simulink model "c_Simulink_Maglev_Tower_lift_motion_control"  (R2020a)
settings: Solver=ode1  StartTime=0.0  StopTime=1  FixedStep=dt  RelTol=1e-3
InitFcn:
  | %parameters_Maglev_Tower_lift_motion
values from neighbouring files (symbols this model uses):
  A1 = -2*r*cos(w0)    [a_system_response_continuous.m]    (also in a_system_response_discrete.m; b_parameters_Maglev_Tower_lift_motion.m)
  A2 = r*r    (= 0.9801)    [a_system_response_continuous.m]    (also in a_system_response_discrete.m; b_parameters_Maglev_Tower_lift_motion.m)
  b = 2*pi*1    (= 6.28318530718)    [a_system_response_continuous.m]    (also in a_system_response_discrete.m; b_parameters_Maglev_Tower_lift_motion.m = 0)
  B0 = 1    [a_system_response_continuous.m]    (also in a_system_response_discrete.m; b_parameters_Maglev_Tower_lift_motion.m)
  B1 = -2*cos(w0)    [a_system_response_continuous.m]    (also in a_system_response_discrete.m; b_parameters_Maglev_Tower_lift_motion.m)
  B2 = 1    [a_system_response_continuous.m]    (also in a_system_response_discrete.m; b_parameters_Maglev_Tower_lift_motion.m)
  d = dt/(dt+2*tau_current)    (= 0.0591173974417)    [a_system_response_discrete.m]    (also in b_parameters_Maglev_Tower_lift_motion.m = 0.12947)
  dpitch_ref_frequency = 2*pi*0.5    (= 3.14159265359)    [b_parameters_Maglev_Tower_lift_motion.m]
  dpitch_ref_mag = 0.001    [b_parameters_Maglev_Tower_lift_motion.m]
  droll_ref_frequency = 2*pi*0.1    (= 0.628318530718)    [b_parameters_Maglev_Tower_lift_motion.m]
  droll_ref_mag = 0.001    [b_parameters_Maglev_Tower_lift_motion.m]
  dt = 1/5000    (= 0.0002)    [a_system_response_discrete.m]    (also in b_parameters_Maglev_Tower_lift_motion.m)
  dx_ref_frequency = 2*pi*5    (= 31.4159265359)    [b_parameters_Maglev_Tower_lift_motion.m]
  dx_ref_mag = 0.001    [b_parameters_Maglev_Tower_lift_motion.m]
  dy_ref_frequency = 2*pi*10    (= 62.8318530718)    [b_parameters_Maglev_Tower_lift_motion.m]
  dy_ref_mag = 0.001    [b_parameters_Maglev_Tower_lift_motion.m]
  dyaw_ref_frequency = 2*pi*1    (= 6.28318530718)    [b_parameters_Maglev_Tower_lift_motion.m]
  dyaw_ref_mag = 0.001    [b_parameters_Maglev_Tower_lift_motion.m]
  h = 327.07 * 1e-3    (= 0.32707)    [b_parameters_Maglev_Tower_lift_motion.m]
  ha = 373.57 * 1e-3    (= 0.37357)    [b_parameters_Maglev_Tower_lift_motion.m]
  isnoise = 1    [b_parameters_Maglev_Tower_lift_motion.m]
  Ix = Ix_cg    (= 41.394)    [b_parameters_Maglev_Tower_lift_motion.m]
  Iy = Iy_cg + M*da^2    (= 47.4067057344)    [b_parameters_Maglev_Tower_lift_motion.m]
  Iz = Iz_cg + M*da^2    (= 31.5217057344)    [b_parameters_Maglev_Tower_lift_motion.m]
  kc_current = 1    [b_parameters_Maglev_Tower_lift_motion.m]
  ki_current = 1    [b_parameters_Maglev_Tower_lift_motion.m]
  ki_pitch = ki    (= 500)    [b_parameters_Maglev_Tower_lift_motion.m]    (also in c_main_Maglev_Tower_lift_motion_control.m = ki_pitch*dt)
  ki_roll = ki    (= 500)    [b_parameters_Maglev_Tower_lift_motion.m]    (also in c_main_Maglev_Tower_lift_motion_control.m = ki_roll*dt)
  ki_x = ki    (= 500)    [b_parameters_Maglev_Tower_lift_motion.m]    (also in c_main_Maglev_Tower_lift_motion_control.m = ki_x*dt)
  ki_y = ki    (= 500)    [b_parameters_Maglev_Tower_lift_motion.m]    (also in c_main_Maglev_Tower_lift_motion_control.m = ki_y*dt)
  ki_yaw = ki    (= 500)    [b_parameters_Maglev_Tower_lift_motion.m]    (also in c_main_Maglev_Tower_lift_motion_control.m = ki_yaw*dt)
  kp_pitch = kp    (= 0.5)    [b_parameters_Maglev_Tower_lift_motion.m]    (also in c_main_Maglev_Tower_lift_motion_control.m = kp_pitch*dt)
  kp_roll = kp    (= 0.5)    [b_parameters_Maglev_Tower_lift_motion.m]    (also in c_main_Maglev_Tower_lift_motion_control.m = kp_roll*dt)
  kp_x = kp    (= 0.5)    [b_parameters_Maglev_Tower_lift_motion.m]    (also in c_main_Maglev_Tower_lift_motion_control.m = kp_x*dt)
  kp_y = kp    (= 0.5)    [b_parameters_Maglev_Tower_lift_motion.m]    (also in c_main_Maglev_Tower_lift_motion_control.m = kp_y*dt)
  kp_yaw = kp    (= 0.5)    [b_parameters_Maglev_Tower_lift_motion.m]    (also in c_main_Maglev_Tower_lift_motion_control.m = kp_yaw*dt)
  M = 302.667    [b_parameters_Maglev_Tower_lift_motion.m]
  pBu = pinv(Bu)    [b_parameters_Maglev_Tower_lift_motion.m]
  select_current_filter = 3    [b_parameters_Maglev_Tower_lift_motion.m]
  tau = 1/(2*pi*100)    (= 0.00159154943092)    [a_system_response_continuous.m]    (also in a_system_response_discrete.m; b_parameters_Maglev_Tower_lift_motion.m)
  tau_current = 1/(2*pi*100)    (= 0.00159154943092)    [a_system_response_continuous.m]    (also in a_system_response_discrete.m; b_parameters_Maglev_Tower_lift_motion.m)
  w = 219.77 * 1e-3    (= 0.21977)    [b_parameters_Maglev_Tower_lift_motion.m]
  w_current = 2*pi*5    (= 31.4159265359)    [a_system_response_continuous.m]    (also in a_system_response_discrete.m; b_parameters_Maglev_Tower_lift_motion.m)
  wa = 140.52 * 1e-3    (= 0.14052)    [b_parameters_Maglev_Tower_lift_motion.m]
  zeta = 0.707    [a_system_response_continuous.m]    (also in a_system_response_discrete.m; b_parameters_Maglev_Tower_lift_motion.m)
libraries: simulink x8
settings Model: Creator=JSPark  LastModifiedBy=JSPark
settings SolverCC: AlgebraicLoopSolver=LineSearch

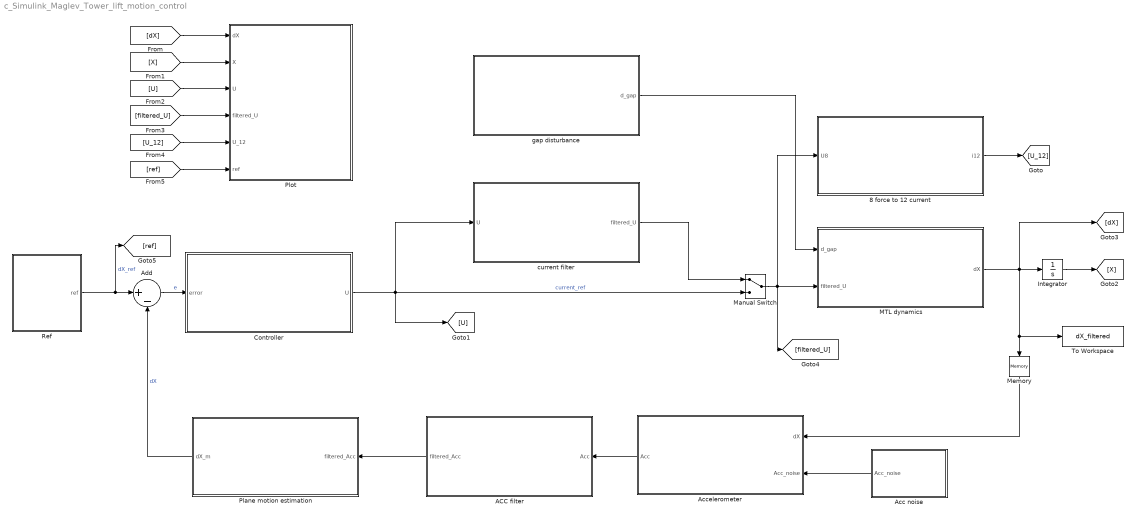
== system c_Simulink_Maglev_Tower_lift_motion_control ==
  8 force to 12 current : Subsystem
  ACC filter : Subsystem
  Acc noise : Subsystem
  Accelerometer : Subsystem
  Add : Sum  Inputs=|+-
  Controller : Subsystem
  Integrator : Integrator
  MTL dynamics : Subsystem
  Manual Switch : ManualSwitch
  Memory : Memory
  Plane motion estimation : Subsystem
  Plot : Subsystem
  Ref : Subsystem
  To Workspace : ToWorkspace  VariableName=dX_filtered  SampleTime=-1
  current filter : Subsystem
  gap disturbance : Subsystem
  wires:
  MTL dynamics/1(dX) -> [dX], To Workspace/1, Memory/1, Integrator/1
  Ref/1(ref) -> [ref], Add/1  "dX_ref"
  Plane motion estimation/1(dX_m) -> Add/2  "dX"
  Add/1 -> Controller/1(error)  "e"
  Accelerometer/1(Acc) -> ACC filter/1(Acc)
  Memory/1 -> Accelerometer/1(dX)
  Acc noise/1(Acc_noise) -> Accelerometer/2(Acc_noise)
  ACC filter/1(filtered_Acc) -> Plane motion estimation/1(filtered_Acc)
  Controller/1(U) -> [U], Manual Switch/2, current filter/1(U)  "current_ref"
  gap disturbance/1(d_gap) -> MTL dynamics/1(d_gap)
  Manual Switch/1 -> 8 force to 12 current/1(U8), [filtered_U], MTL dynamics/2(filtered_U)
  current filter/1(filtered_U) -> Manual Switch/1
  8 force to 12 current/1(i12) -> [U_12]
  Integrator/1 -> [X]
  [dX] -> Plot/1(dX)
  [X] -> Plot/2(X)
  [U] -> Plot/3(U)
  [filtered_U] -> Plot/4(filtered_U)
  [U_12] -> Plot/5(U_12)
  [ref] -> Plot/6(ref)

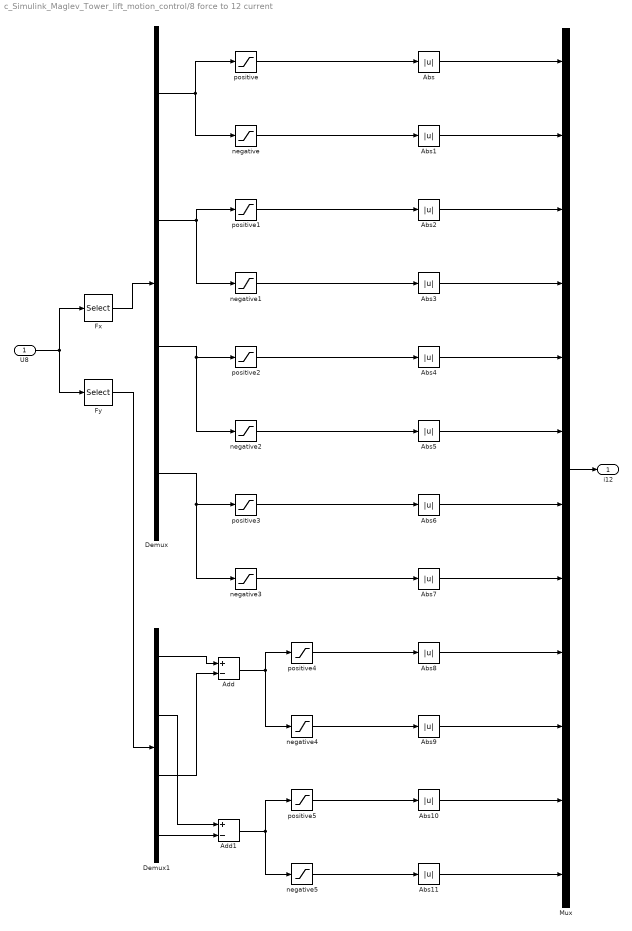
== system c_Simulink_Maglev_Tower_lift_motion_control/8 force to 12 current ==
  U8 : Inport
  Abs{,1..11} (12 alike) : Abs
  Add : Sum  Inputs=+-
  Add1 : Sum  Inputs=+-
  Demux : Demux
  Demux1 : Demux
  Fx : Selector  InputPortWidth=8  IndexOptions=Index vector (dialog)  Indices=[1:4]  OutputSizes=1
  Fy : Selector  InputPortWidth=8  IndexOptions=Index vector (dialog)  Indices=[5:8]  OutputSizes=1
  Mux : Mux  Inputs=12
  negative{,1..5} (6 alike) : Saturate  UpperLimit=0  LowerLimit=-100000
  positive{,1..5} (6 alike) : Saturate  UpperLimit=100000  LowerLimit=0
  i12 : Outport
  wires:
  U8/1 -> Fy/1, Fx/1
  Fx/1 -> Demux/1
  Demux/1 -> negative/1, positive/1
  positive/1 -> Abs/1
  negative/1 -> Abs1/1
  Demux/2 -> negative1/1, positive1/1
  positive1/1 -> Abs2/1
  negative1/1 -> Abs3/1
  positive2/1 -> Abs4/1
  negative2/1 -> Abs5/1
  positive3/1 -> Abs6/1
  negative3/1 -> Abs7/1
  Demux/3 -> negative2/1, positive2/1
  Demux/4 -> positive3/1, negative3/1
  Fy/1 -> Demux1/1
  Demux1/1 -> Add/1
  Demux1/3 -> Add/2
  Demux1/2 -> Add1/1
  Demux1/4 -> Add1/2
  Add/1 -> positive4/1, negative4/1
  Add1/1 -> positive5/1, negative5/1
  positive4/1 -> Abs8/1
  negative4/1 -> Abs9/1
  positive5/1 -> Abs10/1
  negative5/1 -> Abs11/1
  Mux/1 -> i12/1
  Abs/1 -> Mux/1
  Abs1/1 -> Mux/2
  Abs2/1 -> Mux/3
  Abs3/1 -> Mux/4
  Abs4/1 -> Mux/5
  Abs5/1 -> Mux/6
  Abs6/1 -> Mux/7
  Abs7/1 -> Mux/8
  Abs8/1 -> Mux/9
  Abs9/1 -> Mux/10
  Abs10/1 -> Mux/11
  Abs11/1 -> Mux/12

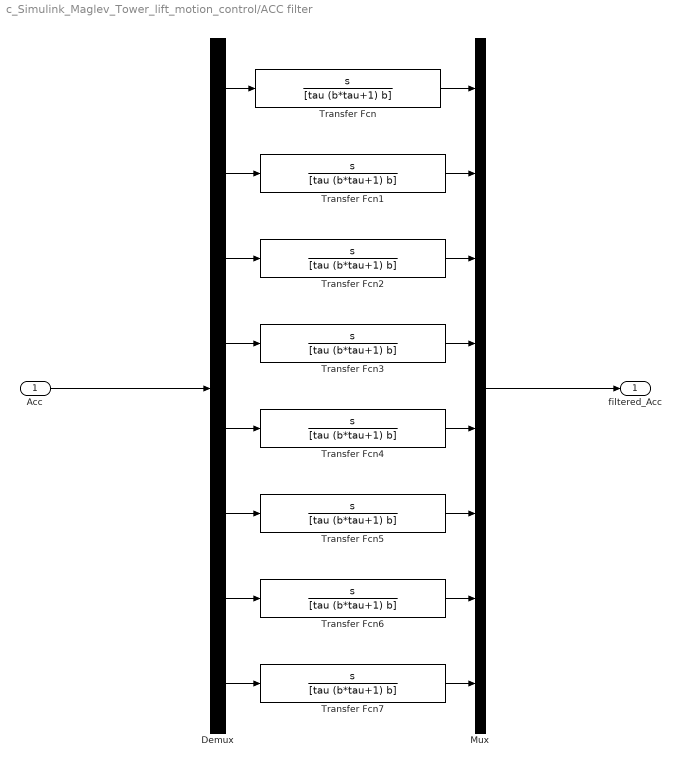
== system c_Simulink_Maglev_Tower_lift_motion_control/ACC filter ==
  Acc : Inport
  Demux : Demux  Outputs=8
  Mux : Mux  Inputs=8
  Transfer Fcn{,1..7} (8 alike) : TransferFcn  Numerator=[1 0]  Denominator=[tau (b*tau+1) b]
  filtered_Acc : Outport
  wires:
  Acc/1 -> Demux/1
  Demux/1 -> Transfer Fcn/1
  Demux/2 -> Transfer Fcn1/1
  Demux/3 -> Transfer Fcn2/1
  Demux/4 -> Transfer Fcn3/1
  Demux/5 -> Transfer Fcn4/1
  Demux/6 -> Transfer Fcn5/1
  Demux/7 -> Transfer Fcn6/1
  Demux/8 -> Transfer Fcn7/1
  Transfer Fcn/1 -> Mux/1
  Transfer Fcn1/1 -> Mux/2
  Transfer Fcn2/1 -> Mux/3
  Transfer Fcn3/1 -> Mux/4
  Transfer Fcn4/1 -> Mux/5
  Transfer Fcn5/1 -> Mux/6
  Transfer Fcn6/1 -> Mux/7
  Transfer Fcn7/1 -> Mux/8
  Mux/1 -> filtered_Acc/1

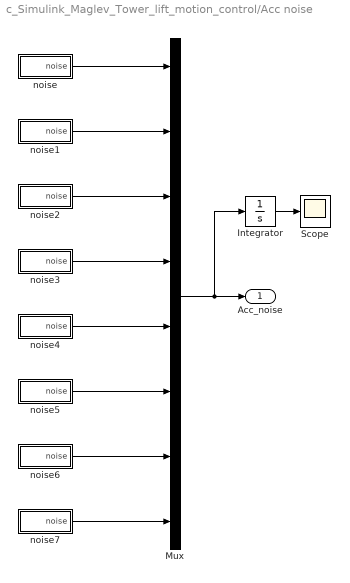
== system c_Simulink_Maglev_Tower_lift_motion_control/Acc noise ==
  Integrator : Integrator
  Mux : Mux  Inputs=8
  Scope : Scope
  noise : Subsystem
  noise1 : Subsystem
  noise2 : Subsystem
  noise3 : Subsystem
  noise4 : Subsystem
  noise5 : Subsystem
  noise6 : Subsystem
  noise7 : Subsystem
  Acc_noise : Outport
  wires:
  noise3/1(noise) -> Mux/4
  noise6/1(noise) -> Mux/7
  noise5/1(noise) -> Mux/6
  noise7/1(noise) -> Mux/8
  noise2/1(noise) -> Mux/3
  noise1/1(noise) -> Mux/2
  noise/1(noise) -> Mux/1
  noise4/1(noise) -> Mux/5
  Mux/1 -> Integrator/1, Acc_noise/1
  Integrator/1 -> Scope/1

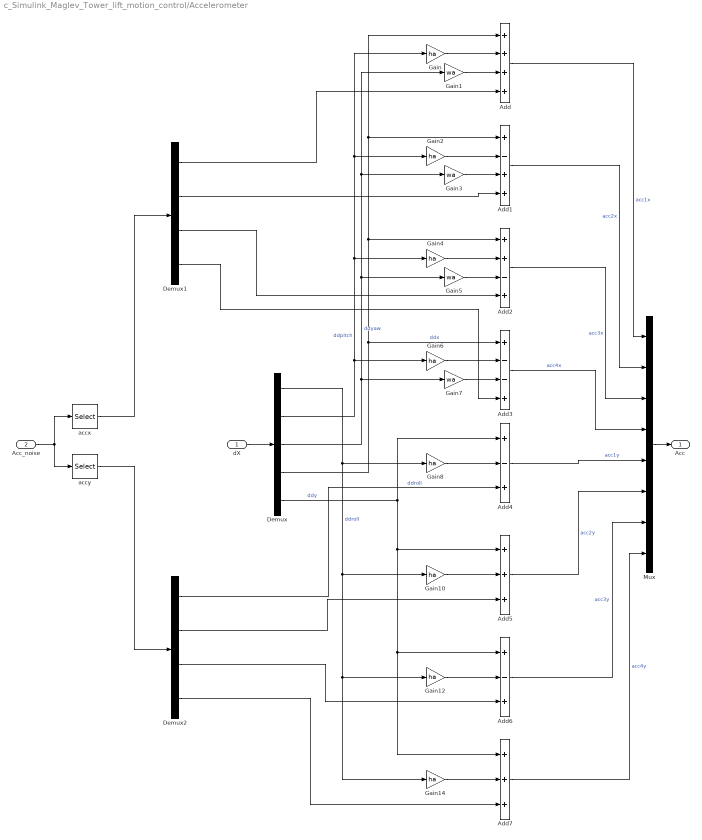
== system c_Simulink_Maglev_Tower_lift_motion_control/Accelerometer ==
  dX : Inport
  Acc_noise : Inport  Port=2
  Add : Sum  Inputs=++++
  Add1 : Sum  Inputs=+-++
  Add2 : Sum  Inputs=++-+
  Add3 : Sum  Inputs=+--+
  Add4 : Sum  Inputs=+-+
  Add5 : Sum  Inputs=+++
  Add6 : Sum  Inputs=+-+
  Add7 : Sum  Inputs=+++
  Demux : Demux  Outputs=5
  Demux1 : Demux
  Demux2 : Demux
  Gain{,2,4,6,8,10,12,14} (8 alike) : Gain  Gain=ha
  Gain{1,3,5,7} (4 alike) : Gain  Gain=wa
  Mux : Mux  Inputs=8
  accx : Selector  InputPortWidth=8  IndexOptions=Index vector (dialog)  Indices=[1:4]  OutputSizes=1
  accy : Selector  InputPortWidth=8  IndexOptions=Index vector (dialog)  Indices=[5:8]  OutputSizes=1
  Acc : Outport
  wires:
  Mux/1 -> Acc/1
  Demux/4 -> Add3/1, Add2/1, Add1/1, Add/1  "ddx"
  Demux/2 -> Gain6/1, Gain4/1, Gain2/1, Gain/1  "ddpitch"
  Demux/3 -> Gain7/1, Gain5/1, Gain3/1, Gain1/1  "ddyaw"
  Gain/1 -> Add/2
  Gain1/1 -> Add/3
  Add/1 -> Mux/1  "acc1x"
  Gain3/1 -> Add1/3
  Gain2/1 -> Add1/2
  Add1/1 -> Mux/2  "acc2x"
  Gain4/1 -> Add2/2
  Gain5/1 -> Add2/3
  Add2/1 -> Mux/3  "acc3x"
  Gain7/1 -> Add3/3
  Gain6/1 -> Add3/2
  Demux1/4 -> Add3/4
  Add3/1 -> Mux/4  "acc4x"
  Gain10/1 -> Add5/2
  Add4/1 -> Mux/5  "acc1y"
  Add7/1 -> Mux/8  "acc4y"
  Add6/1 -> Mux/7  "acc3y"
  Gain12/1 -> Add6/2
  Gain14/1 -> Add7/2
  Add5/1 -> Mux/6  "acc2y"
  Gain8/1 -> Add4/2
  Demux/5 -> Add5/1, Add6/1, Add7/1, Add4/1  "ddy"
  Demux/1 -> Gain8/1, Gain10/1, Gain12/1, Gain14/1  "ddroll"
  Demux2/2 -> Add5/3
  Demux2/3 -> Add6/3
  Demux2/4 -> Add7/3
  dX/1 -> Demux/1
  Acc_noise/1 -> accy/1, accx/1
  Demux1/1 -> Add/4
  Demux1/2 -> Add1/4
  Demux1/3 -> Add2/4
  Demux2/1 -> Add4/3  "ddroll"
  accx/1 -> Demux1/1
  accy/1 -> Demux2/1

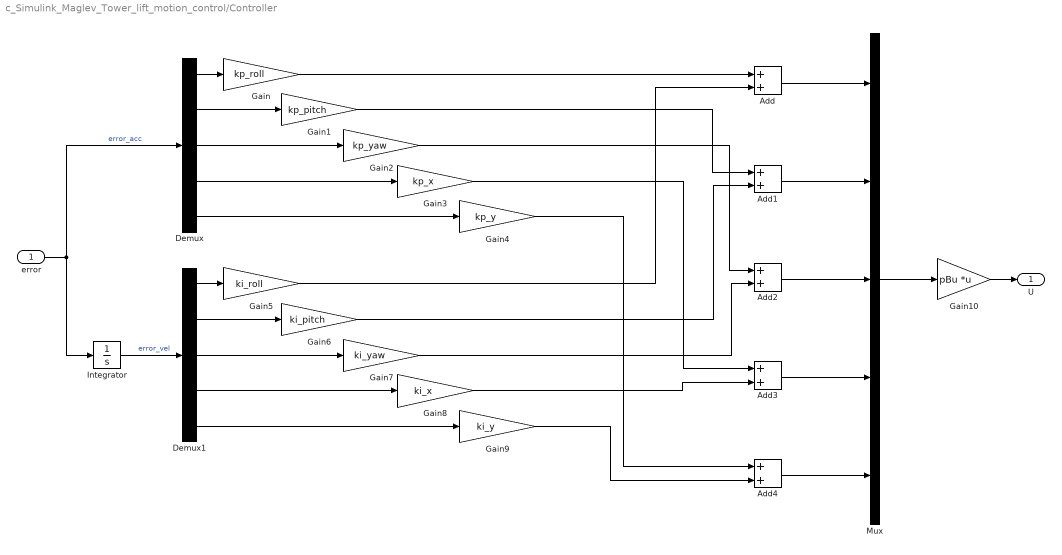
== system c_Simulink_Maglev_Tower_lift_motion_control/Controller ==
  error : Inport
  Add{,1..4} (5 alike) : Sum
  Demux : Demux  Outputs=5
  Demux1 : Demux  Outputs=5
  Gain : Gain  Gain=kp_roll
  Gain1 : Gain  Gain=kp_pitch
  Gain10 : Gain  Gain=pBu  Multiplication=Matrix(K*u)
  Gain2 : Gain  Gain=kp_yaw
  Gain3 : Gain  Gain=kp_x
  Gain4 : Gain  Gain=kp_y
  Gain5 : Gain  Gain=ki_roll
  Gain6 : Gain  Gain=ki_pitch
  Gain7 : Gain  Gain=ki_yaw
  Gain8 : Gain  Gain=ki_x
  Gain9 : Gain  Gain=ki_y
  Integrator : Integrator
  Mux : Mux  Inputs=5
  U : Outport
  wires:
  error/1 -> Integrator/1, Demux/1  "error_acc"
  Integrator/1 -> Demux1/1  "error_vel"
  Demux/1 -> Gain/1
  Demux/2 -> Gain1/1
  Demux/3 -> Gain2/1
  Demux/4 -> Gain3/1
  Demux/5 -> Gain4/1
  Demux1/3 -> Gain7/1
  Demux1/2 -> Gain6/1
  Demux1/5 -> Gain9/1
  Demux1/4 -> Gain8/1
  Demux1/1 -> Gain5/1
  Gain/1 -> Add/1
  Gain5/1 -> Add/2
  Gain1/1 -> Add1/1
  Gain6/1 -> Add1/2
  Gain2/1 -> Add2/1
  Gain7/1 -> Add2/2
  Gain3/1 -> Add3/1
  Gain8/1 -> Add3/2
  Gain4/1 -> Add4/1
  Gain9/1 -> Add4/2
  Add/1 -> Mux/1
  Add1/1 -> Mux/2
  Add2/1 -> Mux/3
  Add3/1 -> Mux/4
  Add4/1 -> Mux/5
  Mux/1 -> Gain10/1
  Gain10/1 -> U/1

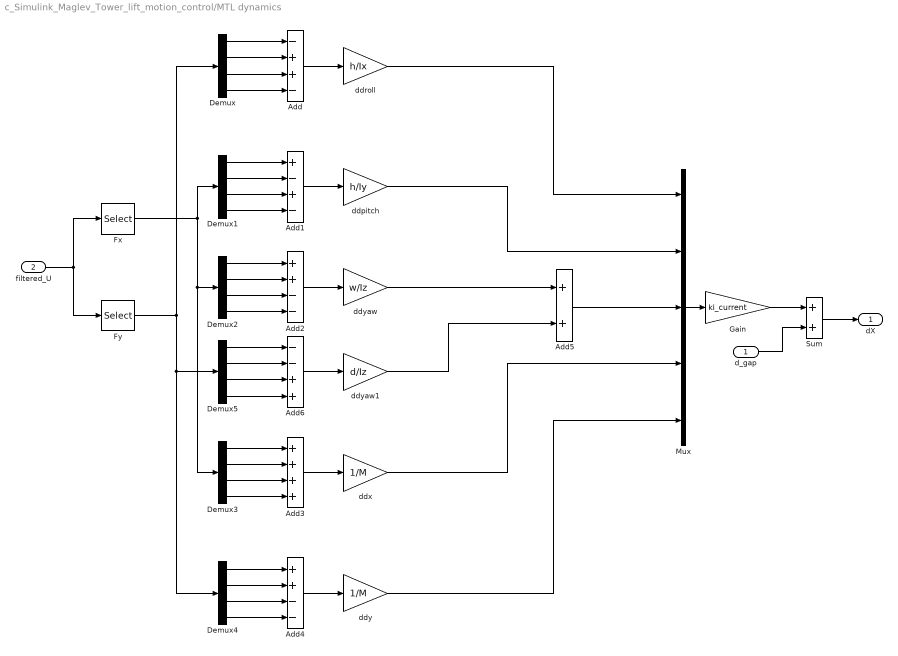
== system c_Simulink_Maglev_Tower_lift_motion_control/MTL dynamics ==
  d_gap : Inport
  filtered_U : Inport  Port=2
  Add : Sum  Inputs=-++-
  Add1 : Sum  Inputs=+-+-
  Add2 : Sum  Inputs=++--
  Add3 : Sum  Inputs=++++
  Add4 : Sum  Inputs=++--
  Add5 : Sum
  Add6 : Sum  Inputs=--++
  Demux{,1..5} (6 alike) : Demux
  Fx : Selector  InputPortWidth=8  IndexOptions=Index vector (dialog)  Indices=[1:4]  OutputSizes=1
  Fy : Selector  InputPortWidth=8  IndexOptions=Index vector (dialog)  Indices=[5:8]  OutputSizes=1
  Gain : Gain  Gain=ki_current
  Mux : Mux  Inputs=5
  Sum : Sum
  ddpitch : Gain  Gain=h/Iy
  ddroll : Gain  Gain=h/Ix
  ddx : Gain  Gain=1/M
  ddy : Gain  Gain=1/M
  ddyaw : Gain  Gain=w/Iz
  ddyaw1 : Gain  Gain=d/Iz
  dX : Outport
  wires:
  Add/1 -> ddroll/1
  filtered_U/1 -> Fy/1, Fx/1
  Demux/1 -> Add/1
  Demux/2 -> Add/2
  Demux/3 -> Add/3
  Demux/4 -> Add/4
  Add1/1 -> ddpitch/1
  Demux1/1 -> Add1/1
  Demux1/3 -> Add1/3
  Demux1/2 -> Add1/2
  Demux1/4 -> Add1/4
  Demux2/4 -> Add2/4
  Demux2/2 -> Add2/2
  Demux2/3 -> Add2/3
  Demux2/1 -> Add2/1
  Add2/1 -> ddyaw/1
  Fx/1 -> Demux3/1, Demux2/1, Demux1/1
  Add3/1 -> ddx/1
  Demux3/1 -> Add3/1
  Demux3/3 -> Add3/3
  Demux3/2 -> Add3/2
  Demux3/4 -> Add3/4
  Demux4/2 -> Add4/2
  Demux4/3 -> Add4/3
  Demux4/1 -> Add4/1
  Add4/1 -> ddy/1
  Demux4/4 -> Add4/4
  Mux/1 -> Gain/1
  ddpitch/1 -> Mux/2
  ddroll/1 -> Mux/1
  ddx/1 -> Mux/4
  ddy/1 -> Mux/5
  Add5/1 -> Mux/3
  ddyaw/1 -> Add5/1
  Demux5/2 -> Add6/2
  Add6/1 -> ddyaw1/1
  Demux5/4 -> Add6/4
  Demux5/3 -> Add6/3
  Demux5/1 -> Add6/1
  ddyaw1/1 -> Add5/2
  Fy/1 -> Demux4/1, Demux5/1, Demux/1
  Gain/1 -> Sum/1
  d_gap/1 -> Sum/2
  Sum/1 -> dX/1

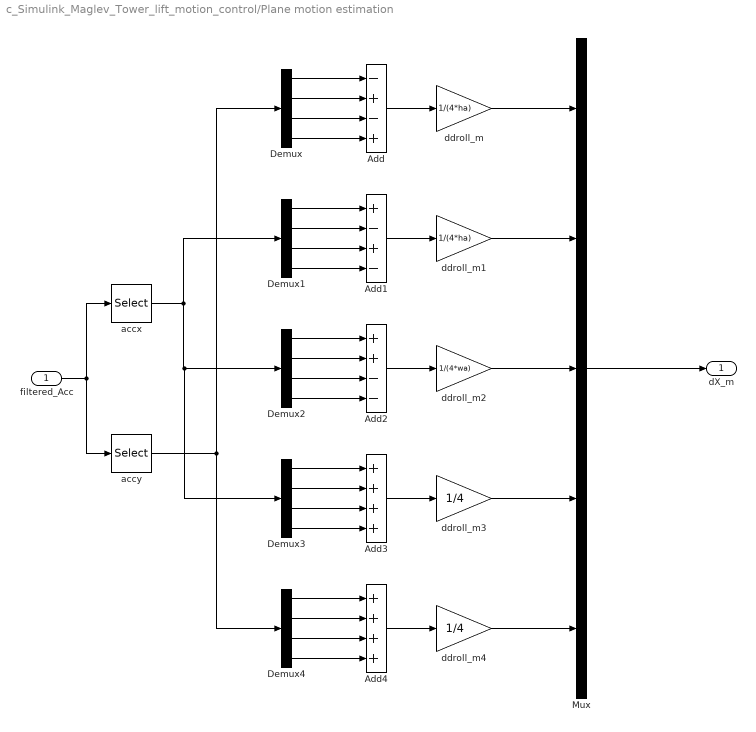
== system c_Simulink_Maglev_Tower_lift_motion_control/Plane motion estimation ==
  filtered_Acc : Inport
  Add : Sum  Inputs=-+-+
  Add1 : Sum  Inputs=+-+-
  Add2 : Sum  Inputs=++--
  Add3 : Sum  Inputs=++++
  Add4 : Sum  Inputs=++++
  Demux{,1..4} (5 alike) : Demux
  Mux : Mux  Inputs=5
  accx : Selector  InputPortWidth=8  IndexOptions=Index vector (dialog)  Indices=[1:4]  OutputSizes=1
  accy : Selector  InputPortWidth=8  IndexOptions=Index vector (dialog)  Indices=[5:8]  OutputSizes=1
  ddroll_m : Gain  Gain=1/(4*ha)
  ddroll_m1 : Gain  Gain=1/(4*ha)
  ddroll_m2 : Gain  Gain=1/(4*wa)
  ddroll_m3 : Gain  Gain=1/4
  ddroll_m4 : Gain  Gain=1/4
  dX_m : Outport
  wires:
  filtered_Acc/1 -> accy/1, accx/1
  Add/1 -> ddroll_m/1
  Demux/1 -> Add/1
  Demux/3 -> Add/3
  Demux/2 -> Add/2
  Demux/4 -> Add/4
  accy/1 -> Demux4/1, Demux/1
  Demux1/4 -> Add1/4
  Demux1/1 -> Add1/1
  Demux1/2 -> Add1/2
  Add1/1 -> ddroll_m1/1
  Demux1/3 -> Add1/3
  accx/1 -> Demux3/1, Demux2/1, Demux1/1
  Demux2/4 -> Add2/4
  Demux2/1 -> Add2/1
  Demux2/2 -> Add2/2
  Add2/1 -> ddroll_m2/1
  Demux2/3 -> Add2/3
  Demux3/4 -> Add3/4
  Demux3/1 -> Add3/1
  Demux3/2 -> Add3/2
  Add3/1 -> ddroll_m3/1
  Demux3/3 -> Add3/3
  Demux4/4 -> Add4/4
  Demux4/1 -> Add4/1
  Demux4/2 -> Add4/2
  Add4/1 -> ddroll_m4/1
  Demux4/3 -> Add4/3
  ddroll_m/1 -> Mux/1
  ddroll_m1/1 -> Mux/2
  ddroll_m2/1 -> Mux/3
  ddroll_m3/1 -> Mux/4
  ddroll_m4/1 -> Mux/5
  Mux/1 -> dX_m/1

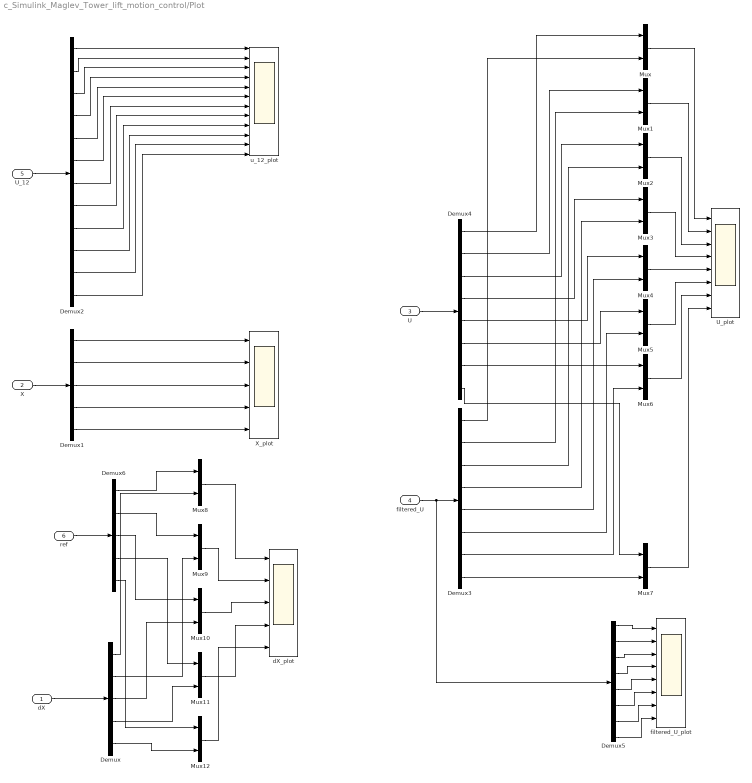
== system c_Simulink_Maglev_Tower_lift_motion_control/Plot ==
  dX : Inport
  X : Inport  Port=2
  U : Inport  Port=3
  filtered_U : Inport  Port=4
  U_12 : Inport  Port=5
  ref : Inport  Port=6
  Demux : Demux  Outputs=5
  Demux1 : Demux  Outputs=5
  Demux2 : Demux  Outputs=12
  Demux3 : Demux  Outputs=8
  Demux4 : Demux  Outputs=8
  Demux5 : Demux  Outputs=8
  Demux6 : Demux  Outputs=5
  Mux{,1..12} (13 alike) : Mux  Inputs=2
  U_plot : Scope  NumInputPorts=8
  X_plot : Scope  NumInputPorts=5
  dX_plot : Scope  NumInputPorts=5
  filtered_U_plot : Scope  NumInputPorts=8
  u_12_plot : Scope  NumInputPorts=12
  wires:
  Mux4/1 -> U_plot/5
  Mux7/1 -> U_plot/8
  Mux5/1 -> U_plot/6
  Demux3/3 -> Mux2/2
  Mux6/1 -> U_plot/7
  Demux4/2 -> Mux1/1
  Mux2/1 -> U_plot/3
  Demux4/8 -> Mux7/1
  Demux4/4 -> Mux3/1
  Mux1/1 -> U_plot/2
  Mux3/1 -> U_plot/4
  Demux3/8 -> Mux7/2
  Demux4/1 -> Mux/1
  Demux4/7 -> Mux6/1
  Demux2/8 -> u_12_plot/8
  Demux2/4 -> u_12_plot/4
  Demux3/7 -> Mux6/2
  Demux3/6 -> Mux5/2
  Demux4/6 -> Mux5/1
  Demux4/5 -> Mux4/1
  Demux2/7 -> u_12_plot/7
  Demux1/5 -> X_plot/5
  Demux2/12 -> u_12_plot/12
  Demux2/2 -> u_12_plot/2
  Demux3/5 -> Mux4/2
  Demux3/4 -> Mux3/2
  Demux4/3 -> Mux2/1
  Demux3/2 -> Mux1/2
  Mux/1 -> U_plot/1
  U_12/1 -> Demux2/1
  X/1 -> Demux1/1
  U/1 -> Demux4/1
  Demux1/4 -> X_plot/4
  Demux2/5 -> u_12_plot/5
  Demux2/10 -> u_12_plot/10
  Demux1/3 -> X_plot/3
  Demux2/9 -> u_12_plot/9
  Demux2/6 -> u_12_plot/6
  Demux2/3 -> u_12_plot/3
  Demux2/11 -> u_12_plot/11
  Demux1/1 -> X_plot/1
  Demux2/1 -> u_12_plot/1
  Demux1/2 -> X_plot/2
  Demux3/1 -> Mux/2
  Demux5/2 -> filtered_U_plot/2
  Demux5/1 -> filtered_U_plot/1
  Demux5/3 -> filtered_U_plot/3
  Demux5/4 -> filtered_U_plot/4
  Demux5/5 -> filtered_U_plot/5
  Demux5/6 -> filtered_U_plot/6
  Demux5/7 -> filtered_U_plot/7
  Demux5/8 -> filtered_U_plot/8
  filtered_U/1 -> Demux5/1, Demux3/1
  ref/1 -> Demux6/1
  Mux8/1 -> dX_plot/1
  Mux9/1 -> dX_plot/2
  Mux10/1 -> dX_plot/3
  Mux11/1 -> dX_plot/4
  Mux12/1 -> dX_plot/5
  dX/1 -> Demux/1
  Demux6/1 -> Mux8/1
  Demux6/2 -> Mux9/1
  Demux6/3 -> Mux10/1
  Demux6/4 -> Mux11/1
  Demux6/5 -> Mux12/1
  Demux/1 -> Mux8/2
  Demux/2 -> Mux9/2
  Demux/3 -> Mux10/2
  Demux/4 -> Mux11/2
  Demux/5 -> Mux12/2

== system c_Simulink_Maglev_Tower_lift_motion_control/Ref ==
  Mux : Mux  Inputs=5
  Sine Wave : Sin  Amplitude=droll_ref_mag  Frequency=droll_ref_frequency  Phase=pi/2  SampleTime=0
  Sine Wave1 : Sin  Amplitude=dpitch_ref_mag  Frequency=dpitch_ref_frequency  Phase=pi/2  SampleTime=0
  Sine Wave2 : Sin  Amplitude=dyaw_ref_mag  Frequency=dyaw_ref_frequency  Phase=pi/2  SampleTime=0
  Sine Wave3 : Sin  Amplitude=dx_ref_mag  Frequency=dx_ref_frequency  Phase=pi/2  SampleTime=0
  Sine Wave4 : Sin  Amplitude=dy_ref_mag  Frequency=dy_ref_frequency  Phase=pi/2  SampleTime=0
  ref : Outport
  wires:
  Mux/1 -> ref/1
  Sine Wave/1 -> Mux/1
  Sine Wave1/1 -> Mux/2
  Sine Wave2/1 -> Mux/3
  Sine Wave3/1 -> Mux/4
  Sine Wave4/1 -> Mux/5

== system c_Simulink_Maglev_Tower_lift_motion_control/current filter ==
  U : Inport
  1st order highpass filter : Subsystem
  2nd order highpass filter : Subsystem
  2nd order highpass filter + 1st order low pass filter : Subsystem
  Constant : Constant  Value=select_current_filter
  Multiport Switch : MultiPortSwitch  Inputs=4
  notch filter (digital IIR filter) : Subsystem
  filtered_U : Outport
  wires:
  U/1 -> 2nd order highpass filter + 1st order low pass filter/1(U), notch filter (digital IIR filter)/1(U), 2nd order highpass filter/1(U), 1st order highpass filter/1(U)
  Multiport Switch/1 -> filtered_U/1
  Constant/1 -> Multiport Switch/1
  1st order highpass filter/1(highpass filter) -> Multiport Switch/2
  2nd order highpass filter/1(highpass filter) -> Multiport Switch/3
  2nd order highpass filter + 1st order low pass filter/1(highpass filter) -> Multiport Switch/4
  notch filter (digital IIR filter)/1(notch filter (50Hz)) -> Multiport Switch/5

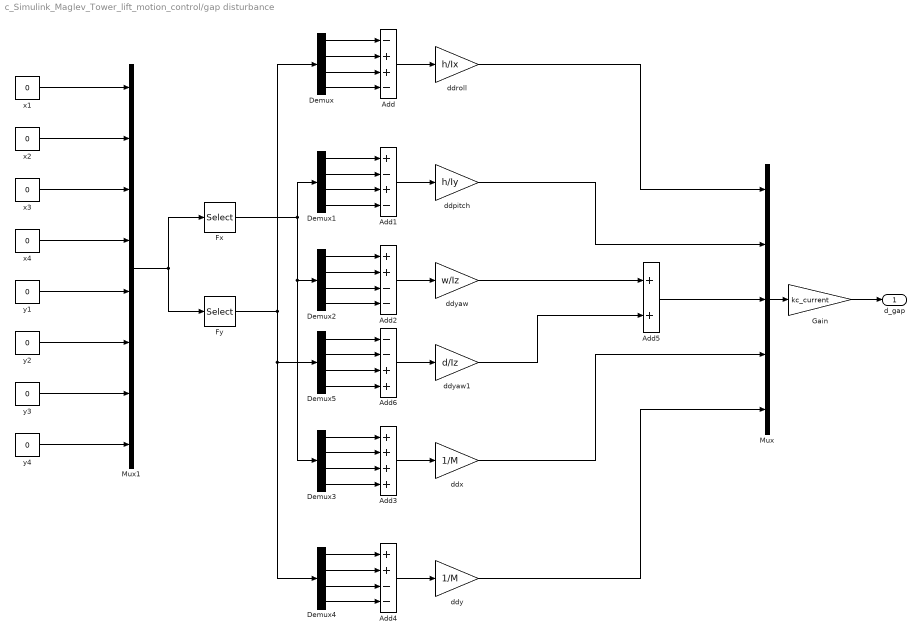
== system c_Simulink_Maglev_Tower_lift_motion_control/gap disturbance ==
  Add : Sum  Inputs=-++-
  Add1 : Sum  Inputs=+-+-
  Add2 : Sum  Inputs=++--
  Add3 : Sum  Inputs=++++
  Add4 : Sum  Inputs=++--
  Add5 : Sum
  Add6 : Sum  Inputs=--++
  Demux{,1..5} (6 alike) : Demux
  Fx : Selector  InputPortWidth=8  IndexOptions=Index vector (dialog)  Indices=[1:4]  OutputSizes=1
  Fy : Selector  InputPortWidth=8  IndexOptions=Index vector (dialog)  Indices=[5:8]  OutputSizes=1
  Gain : Gain  Gain=kc_current
  Mux : Mux  Inputs=5
  Mux1 : Mux  Inputs=8
  ddpitch : Gain  Gain=h/Iy
  ddroll : Gain  Gain=h/Ix
  ddx : Gain  Gain=1/M
  ddy : Gain  Gain=1/M
  ddyaw : Gain  Gain=w/Iz
  ddyaw1 : Gain  Gain=d/Iz
  x{1..4} (4 alike) : Constant  Value=0
  y{1..4} (4 alike) : Constant  Value=0
  d_gap : Outport
  wires:
  ddyaw1/1 -> Add5/2
  Add6/1 -> ddyaw1/1
  Add5/1 -> Mux/3
  ddy/1 -> Mux/5
  Mux/1 -> Gain/1
  ddyaw/1 -> Add5/1
  Add/1 -> ddroll/1
  ddroll/1 -> Mux/1
  ddx/1 -> Mux/4
  Add4/1 -> ddy/1
  ddpitch/1 -> Mux/2
  Add2/1 -> ddyaw/1
  Add3/1 -> ddx/1
  Add1/1 -> ddpitch/1
  Gain/1 -> d_gap/1
  Fx/1 -> Demux3/1, Demux2/1, Demux1/1
  Fy/1 -> Demux4/1, Demux5/1, Demux/1
  x1/1 -> Mux1/1
  x2/1 -> Mux1/2
  x3/1 -> Mux1/3
  x4/1 -> Mux1/4
  y1/1 -> Mux1/5
  y2/1 -> Mux1/6
  y3/1 -> Mux1/7
  y4/1 -> Mux1/8
  Mux1/1 -> Fy/1, Fx/1
  Demux/1 -> Add/1
  Demux/2 -> Add/2
  Demux/3 -> Add/3
  Demux/4 -> Add/4
  Demux1/1 -> Add1/1
  Demux1/2 -> Add1/2
  Demux1/3 -> Add1/3
  Demux1/4 -> Add1/4
  Demux2/1 -> Add2/1
  Demux2/2 -> Add2/2
  Demux2/3 -> Add2/3
  Demux2/4 -> Add2/4
  Demux5/1 -> Add6/1
  Demux5/2 -> Add6/2
  Demux5/3 -> Add6/3
  Demux5/4 -> Add6/4
  Demux3/1 -> Add3/1
  Demux3/2 -> Add3/2
  Demux3/3 -> Add3/3
  Demux3/4 -> Add3/4
  Demux4/1 -> Add4/1
  Demux4/2 -> Add4/2
  Demux4/3 -> Add4/3
  Demux4/4 -> Add4/4

== system c_Simulink_Maglev_Tower_lift_motion_control/Acc noise/noise ==
  Add : Sum  Inputs=+-
  Constant : Constant  Value=0.0005
  Gain : Gain  Gain=0.5
  Gain1 : Gain  Gain=isnoise
  Manual Switch : ManualSwitch
  Normal : RandomNumber  SampleTime=dt
  "Uniform " : UniformRandomNumber  Minimum=0  Maximum=0.001  SampleTime=dt
  noise : Outport
  wires:
  Constant/1 -> Add/2
  Add/1 -> Gain/1
  Gain/1 -> Gain1/1
  Gain1/1 -> noise/1
  Manual Switch/1 -> Add/1
  Normal/1 -> Manual Switch/2
  "Uniform "/1 -> Manual Switch/1

== system c_Simulink_Maglev_Tower_lift_motion_control/Acc noise/noise1 ==
  Add : Sum  Inputs=+-
  Constant : Constant  Value=0.0005
  Gain : Gain  Gain=0.5
  Gain1 : Gain  Gain=isnoise
  Manual Switch : ManualSwitch
  Normal : RandomNumber  Seed=1  SampleTime=dt
  "Uniform " : UniformRandomNumber  Minimum=0  Maximum=0.001  Seed=1  SampleTime=dt
  noise : Outport
  wires:
  Manual Switch/1 -> Add/1
  Constant/1 -> Add/2
  Add/1 -> Gain/1
  Gain/1 -> Gain1/1
  Gain1/1 -> noise/1
  Normal/1 -> Manual Switch/2
  "Uniform "/1 -> Manual Switch/1

== system c_Simulink_Maglev_Tower_lift_motion_control/Acc noise/noise2 ==
  Add : Sum  Inputs=+-
  Constant : Constant  Value=0.0005
  Gain : Gain  Gain=0.5
  Gain1 : Gain  Gain=isnoise
  Manual Switch : ManualSwitch
  Normal : RandomNumber  Seed=2  SampleTime=dt
  "Uniform " : UniformRandomNumber  Minimum=0  Maximum=0.001  Seed=2  SampleTime=dt
  noise : Outport
  wires:
  Manual Switch/1 -> Add/1
  Constant/1 -> Add/2
  Add/1 -> Gain/1
  Gain/1 -> Gain1/1
  Gain1/1 -> noise/1
  Normal/1 -> Manual Switch/2
  "Uniform "/1 -> Manual Switch/1

== system c_Simulink_Maglev_Tower_lift_motion_control/Acc noise/noise3 ==
  Add : Sum  Inputs=+-
  Constant : Constant  Value=0.0005
  Gain : Gain  Gain=0.5
  Gain1 : Gain  Gain=isnoise
  Manual Switch : ManualSwitch
  Normal : RandomNumber  Seed=3  SampleTime=dt
  "Uniform " : UniformRandomNumber  Minimum=0  Maximum=0.001  Seed=3  SampleTime=dt
  noise : Outport
  wires:
  Manual Switch/1 -> Add/1
  Constant/1 -> Add/2
  Add/1 -> Gain/1
  Gain/1 -> Gain1/1
  Gain1/1 -> noise/1
  Normal/1 -> Manual Switch/2
  "Uniform "/1 -> Manual Switch/1

== system c_Simulink_Maglev_Tower_lift_motion_control/Acc noise/noise4 ==
  Add : Sum  Inputs=+-
  Constant : Constant  Value=0.0005
  Gain : Gain  Gain=0.5
  Gain1 : Gain  Gain=isnoise
  Manual Switch : ManualSwitch
  Normal : RandomNumber  Seed=4  SampleTime=dt
  "Uniform " : UniformRandomNumber  Minimum=0  Maximum=0.001  Seed=4  SampleTime=dt
  noise : Outport
  wires:
  Manual Switch/1 -> Add/1
  Constant/1 -> Add/2
  Add/1 -> Gain/1
  Gain/1 -> Gain1/1
  Gain1/1 -> noise/1
  Normal/1 -> Manual Switch/2
  "Uniform "/1 -> Manual Switch/1

== system c_Simulink_Maglev_Tower_lift_motion_control/Acc noise/noise5 ==
  Add : Sum  Inputs=+-
  Constant : Constant  Value=0.0005
  Gain : Gain  Gain=0.5
  Gain1 : Gain  Gain=isnoise
  Manual Switch : ManualSwitch
  Normal : RandomNumber  Seed=5  SampleTime=dt
  "Uniform " : UniformRandomNumber  Minimum=0  Maximum=0.001  Seed=5  SampleTime=dt
  noise : Outport
  wires:
  Manual Switch/1 -> Add/1
  Constant/1 -> Add/2
  Add/1 -> Gain/1
  Gain/1 -> Gain1/1
  Gain1/1 -> noise/1
  Normal/1 -> Manual Switch/2
  "Uniform "/1 -> Manual Switch/1

== system c_Simulink_Maglev_Tower_lift_motion_control/Acc noise/noise6 ==
  Add : Sum  Inputs=+-
  Constant : Constant  Value=0.0005
  Gain : Gain  Gain=0.5
  Gain1 : Gain  Gain=isnoise
  Manual Switch : ManualSwitch
  Normal : RandomNumber  Seed=6  SampleTime=dt
  "Uniform " : UniformRandomNumber  Minimum=0  Maximum=0.001  Seed=6  SampleTime=dt
  noise : Outport
  wires:
  Manual Switch/1 -> Add/1
  Constant/1 -> Add/2
  Add/1 -> Gain/1
  Gain/1 -> Gain1/1
  Gain1/1 -> noise/1
  Normal/1 -> Manual Switch/2
  "Uniform "/1 -> Manual Switch/1

== system c_Simulink_Maglev_Tower_lift_motion_control/Acc noise/noise7 ==
  Add : Sum  Inputs=+-
  Constant : Constant  Value=0.0005
  Gain : Gain  Gain=0.5
  Gain1 : Gain  Gain=isnoise
  Manual Switch : ManualSwitch
  Normal : RandomNumber  Seed=7  SampleTime=dt
  "Uniform " : UniformRandomNumber  Minimum=0  Maximum=0.001  Seed=7  SampleTime=dt
  noise : Outport
  wires:
  Manual Switch/1 -> Add/1
  Constant/1 -> Add/2
  Add/1 -> Gain/1
  Gain/1 -> Gain1/1
  Gain1/1 -> noise/1
  Normal/1 -> Manual Switch/2
  "Uniform "/1 -> Manual Switch/1

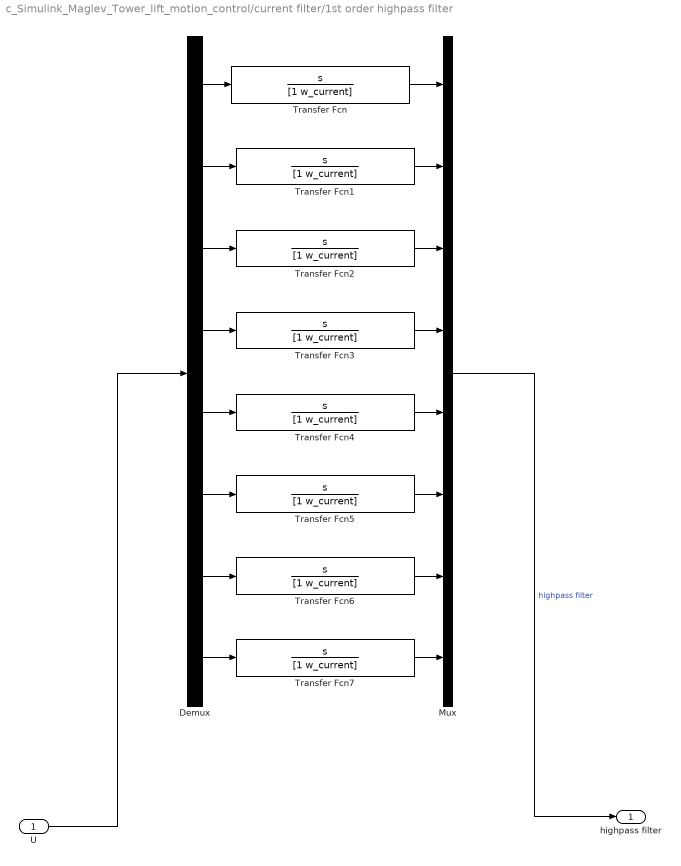
== system c_Simulink_Maglev_Tower_lift_motion_control/current filter/1st order highpass filter ==
  U : Inport
  Demux : Demux  Outputs=8
  Mux : Mux  Inputs=8
  Transfer Fcn{,1..7} (8 alike) : TransferFcn  Numerator=[1 0]  Denominator=[1 w_current]
  highpass filter : Outport
  wires:
  Demux/7 -> Transfer Fcn6/1
  Transfer Fcn2/1 -> Mux/3
  Demux/1 -> Transfer Fcn/1
  Transfer Fcn1/1 -> Mux/2
  Transfer Fcn6/1 -> Mux/7
  Transfer Fcn4/1 -> Mux/5
  Transfer Fcn3/1 -> Mux/4
  Demux/2 -> Transfer Fcn1/1
  Demux/4 -> Transfer Fcn3/1
  Demux/6 -> Transfer Fcn5/1
  Demux/8 -> Transfer Fcn7/1
  Transfer Fcn/1 -> Mux/1
  Transfer Fcn7/1 -> Mux/8
  Demux/3 -> Transfer Fcn2/1
  Transfer Fcn5/1 -> Mux/6
  Demux/5 -> Transfer Fcn4/1
  U/1 -> Demux/1
  Mux/1 -> highpass filter/1  "highpass filter"

== system c_Simulink_Maglev_Tower_lift_motion_control/current filter/2nd order highpass filter ==
  U : Inport
  Demux : Demux  Outputs=8
  Mux : Mux  Inputs=8
  Transfer Fcn{,1..7} (8 alike) : TransferFcn  Numerator=[1 0 0]  Denominator=[1 2*zeta*w_current w_current^2]
  highpass filter : Outport
  wires:
  Demux/7 -> Transfer Fcn6/1
  Demux/1 -> Transfer Fcn/1
  Demux/2 -> Transfer Fcn1/1
  Demux/4 -> Transfer Fcn3/1
  Demux/6 -> Transfer Fcn5/1
  Demux/8 -> Transfer Fcn7/1
  Transfer Fcn/1 -> Mux/1
  Demux/3 -> Transfer Fcn2/1
  Demux/5 -> Transfer Fcn4/1
  U/1 -> Demux/1
  Mux/1 -> highpass filter/1  "highpass filter"
  Transfer Fcn1/1 -> Mux/2
  Transfer Fcn2/1 -> Mux/3
  Transfer Fcn3/1 -> Mux/4
  Transfer Fcn4/1 -> Mux/5
  Transfer Fcn5/1 -> Mux/6
  Transfer Fcn6/1 -> Mux/7
  Transfer Fcn7/1 -> Mux/8

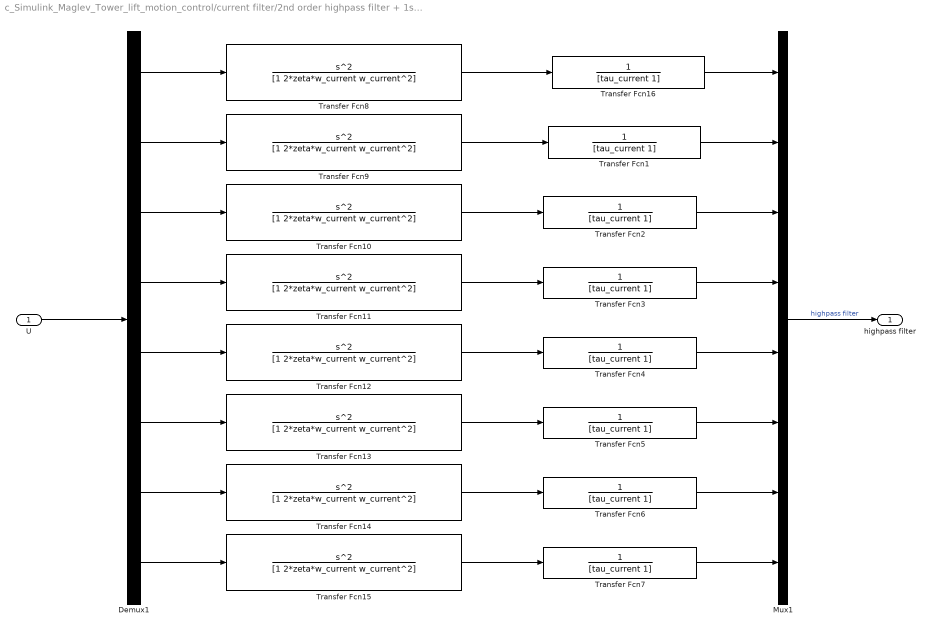
== system c_Simulink_Maglev_Tower_lift_motion_control/current filter/2nd order highpass filter + 1st order low pass filter ==
  U : Inport
  Demux1 : Demux  Outputs=8
  Mux1 : Mux  Inputs=8
  Transfer Fcn{1..7,16} (8 alike) : TransferFcn  Denominator=[tau_current 1]
  Transfer Fcn{8..15} (8 alike) : TransferFcn  Numerator=[1 0 0]  Denominator=[1 2*zeta*w_current w_current^2]
  highpass filter : Outport
  wires:
  Demux1/7 -> Transfer Fcn14/1
  Demux1/4 -> Transfer Fcn11/1
  Demux1/8 -> Transfer Fcn15/1
  Transfer Fcn10/1 -> Transfer Fcn2/1
  Demux1/2 -> Transfer Fcn9/1
  Transfer Fcn9/1 -> Transfer Fcn1/1
  Transfer Fcn11/1 -> Transfer Fcn3/1
  Demux1/1 -> Transfer Fcn8/1
  U/1 -> Demux1/1
  Demux1/5 -> Transfer Fcn12/1
  Transfer Fcn12/1 -> Transfer Fcn4/1
  Demux1/6 -> Transfer Fcn13/1
  Transfer Fcn8/1 -> Transfer Fcn16/1
  Demux1/3 -> Transfer Fcn10/1
  Transfer Fcn13/1 -> Transfer Fcn5/1
  Transfer Fcn14/1 -> Transfer Fcn6/1
  Transfer Fcn15/1 -> Transfer Fcn7/1
  Transfer Fcn16/1 -> Mux1/1
  Mux1/1 -> highpass filter/1  "highpass filter"
  Transfer Fcn1/1 -> Mux1/2
  Transfer Fcn2/1 -> Mux1/3
  Transfer Fcn3/1 -> Mux1/4
  Transfer Fcn4/1 -> Mux1/5
  Transfer Fcn5/1 -> Mux1/6
  Transfer Fcn6/1 -> Mux1/7
  Transfer Fcn7/1 -> Mux1/8

== system c_Simulink_Maglev_Tower_lift_motion_control/current filter/notch filter (digital IIR filter) ==
  U : Inport
  Demux1 : Demux  Outputs=8
  Mux1 : Mux  Inputs=8
  Transfer Fcn Direct Form II{,1..7} (8 alike) : simulink/Additional Math & Discrete/Additional Discrete/Transfer Fcn Direct Form II  NumCoefVec=[B0 B1 B2]  DenCoefVec=[A1 A2]  vinit=0.0  DoSatur=off
      settings: SourceProductBaseCode=SL
  notch filter (50Hz) : Outport
  wires:
  Demux1/8 -> Transfer Fcn Direct Form II7/1
  Transfer Fcn Direct Form II6/1 -> Mux1/7
  Demux1/3 -> Transfer Fcn Direct Form II2/1
  Transfer Fcn Direct Form II3/1 -> Mux1/4
  Demux1/7 -> Transfer Fcn Direct Form II6/1
  Transfer Fcn Direct Form II/1 -> Mux1/1
  Demux1/4 -> Transfer Fcn Direct Form II3/1
  Transfer Fcn Direct Form II1/1 -> Mux1/2
  Demux1/2 -> Transfer Fcn Direct Form II1/1
  Transfer Fcn Direct Form II5/1 -> Mux1/6
  Demux1/6 -> Transfer Fcn Direct Form II5/1
  Mux1/1 -> notch filter (50Hz)/1  "notch filter (50Hz)"
  Transfer Fcn Direct Form II4/1 -> Mux1/5
  Transfer Fcn Direct Form II7/1 -> Mux1/8
  Demux1/5 -> Transfer Fcn Direct Form II4/1
  Transfer Fcn Direct Form II2/1 -> Mux1/3
  Demux1/1 -> Transfer Fcn Direct Form II/1
  U/1 -> Demux1/1
